simulink model "throttle_simulation"  (Simulink 5.0)
settings: Solver=ode45  StartTime=-.25  StopTime=.5-.001  FixedStep=.001  RelTol=1e-3
PreLoadFcn:
  | throttle_simulation_init
StopFcn:
  | throttle_simulation_stopfcn1run
values from neighbouring files (symbols this model uses):
  angle_init = .2    (= 0.2)    [throttle_simulation_init.m]    (also in throttle_simulation_validate.m = mean(position(1:100)) / 90)
  angle_maxopen = 1    [throttle_simulation_init.m]    (also in throttle_simulation_validate.m = max(position)/ 90)
  angle_open = 1    [throttle_simulation_init.m]    (also in throttle_simulation_validate.m = mean(position(end-100:end)) / 90)
  c = 11    [throttle_simulation_init.m]
  k = 1    [throttle_simulation_init.m]
  m = .35    (= 0.35)    [throttle_simulation_init.m]
settings Model: Creator=shirsch  LastModifiedBy=shirsch  SaveTime=off  SaveOutput=off  OutputSaveName=position_s  LimitDataPoints=off  BooleanDataType=off  RTWOptions="-aEnforceIntegerDowncast=1 -aExtMode=0 -aFoldNonRolledExpr=1 -aForceParamTrailComments=0 -aGenerateComments=1 -aIgnoreCustomStorageClasses=1 -aIncHierarchyInIds=0 -aInlineInvariantSignals=0 -aLocalBlockOutputs=1 -aLogVarNameModifier=\"rt_\" -aRTWVerbose=1 -aRollThreshold=5 -aShowEliminatedStatements=1"

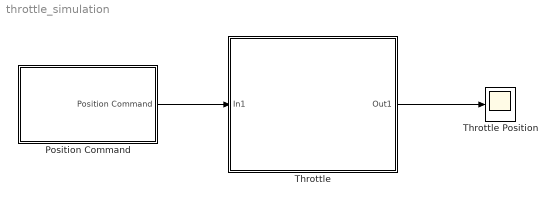
== system throttle_simulation ==
  Position Command : Subsystem
      mask Display: plot([0 1 1 2],[0 0 1 1])
  Throttle : Subsystem  mask{m=m, c=c, k=k, init=angle_init, open=angle_open, upper=angle_maxopen}
      mask prompts: m "Mass"; c "Damping"; k "Stiffness"; init "Resting Angle"; open "Open Angle"; upper "Maximum Open Angle"
      mask init:
      | throttle = imread('Throttle.jpg');
      mask Display: image(throttle)
  Throttle Position : Scope
      settings: TimeRange=0.8  YMin=10  YMax=100  SampleInput=on  SampleTime=0.001
  wires:
  Position Command/1(Position Command) -> Throttle/1(In1)
  Throttle/1(Out1) -> Throttle Position/1

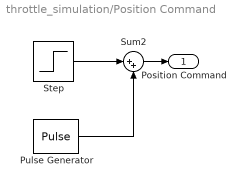
== system throttle_simulation/Position Command ==
  Pulse Generator : DiscretePulseGenerator  PulseType=Time based  Amplitude=-k*(angle_open - angle_init)*.35  Period=100  PulseWidth=.01  PhaseDelay=-.12
  Step : Step  Time=-.11  After=k*(angle_open-angle_init)  SampleTime=0
  Sum2 : Sum  Inputs=|++  SaturateOnIntegerOverflow=on  InputSameDT=on
  Position Command : Outport
  wires:
  Step/1 -> Sum2/1
  Pulse Generator/1 -> Sum2/2
  Sum2/1 -> Position Command/1

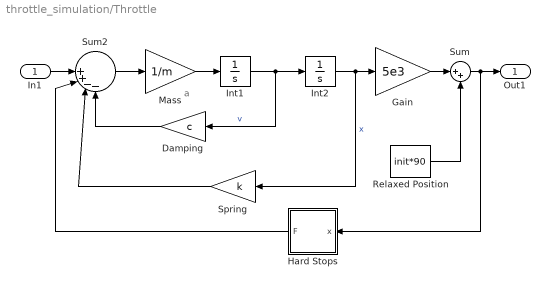
== system throttle_simulation/Throttle ==
  note: a
  In1 : Inport
  Damping : Gain  Orientation=left  Gain=c  SaturateOnIntegerOverflow=on
  Gain : Gain  Gain=5e3  SaturateOnIntegerOverflow=on
  Hard Stops : Subsystem  Orientation=left  mask{H=upper*90, K=5e3, L=init*90}
      mask prompts: H "Upper Limit"; K "Stiffness"; L "Lower Limit"
  Int1 : Integrator
  Int2 : Integrator
  Mass : Gain  Gain=1/m  SaturateOnIntegerOverflow=on
  Relaxed Position : Constant  Value=init*90
  Spring : Gain  Orientation=left  Gain=k  SaturateOnIntegerOverflow=on
  Sum : Sum  Inputs=|++  SaturateOnIntegerOverflow=on  InputSameDT=on
  Sum2 : Sum  Inputs=|||++--  SaturateOnIntegerOverflow=on  InputSameDT=on
  Out1 : Outport
  wires:
  Hard Stops/1(F) -> Sum2/2
  Spring/1 -> Sum2/3
  Damping/1 -> Sum2/4
  Int2/1 -> Gain/1, Spring/1  "x"
  Relaxed Position/1 -> Sum/2
  Sum/1 -> Hard Stops/1(x), Out1/1
  Gain/1 -> Sum/1
  Sum2/1 -> Mass/1
  Mass/1 -> Int1/1
  Int1/1 -> Int2/1, Damping/1  "v"
  In1/1 -> Sum2/1

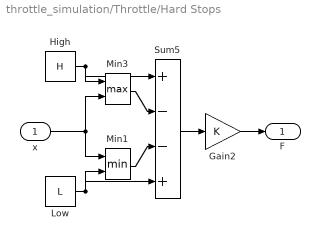
== system throttle_simulation/Throttle/Hard Stops ==
  x : Inport
  Gain2 : Gain  Gain=K  SaturateOnIntegerOverflow=on
  High : Constant  Value=H
  Low : Constant  Value=L
  Min1 : MinMax  Inputs=2
  Min3 : MinMax  Function=max  Inputs=2
  Sum5 : Sum  Inputs=+-||-+  SaturateOnIntegerOverflow=on  InputSameDT=on
  F : Outport
  wires:
  Min1/1 -> Sum5/3
  Min3/1 -> Sum5/2
  High/1 -> Min3/1, Sum5/1
  Low/1 -> Sum5/4, Min1/2
  Sum5/1 -> Gain2/1
  x/1 -> Min3/2, Min1/1
  Gain2/1 -> F/1
